simulink library "icc_lib_avg_path1_n1"  (R2018b)
settings: Solver=VariableStepAuto  StartTime=0.0  StopTime=10.0  RelTol=1e-3
undefined symbols (not defined in the file or in its folder): icc_lib_avg_path, path1
libraries: simulink x34, simulink_extras x8, $bdroot x2
(part 1 of 4)
settings Model: Creator=lwan353  LastModifiedBy=lwan353
settings SFSimCC: SimUseLocalCustomCode=off
settings RTWCC: RTWUseLocalCustomCode=off

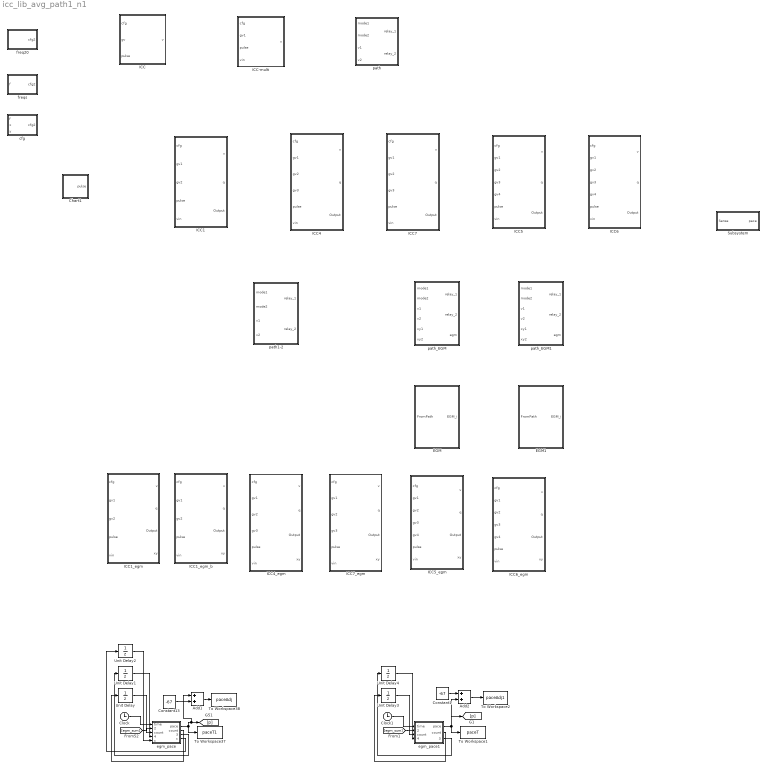
== system icc_lib_avg_path1_n1 ==
  Add1 : Sum
  Add2 : Sum
  Chart1 : Stateflow chart  TreatAsAtomicUnit=on
  Clock : Clock
  Clock1 : Clock
  Constant1 : Constant  Value=-67
  Constant13 : Constant  Value=-67
  EGM : Subsystem
  EGM1 : Subsystem
  "ICC " : Subsystem
  ICC-multi : Subsystem
  ICC1 : Subsystem
  ICC1_egm : Subsystem
  ICC1_egm_b : Subsystem
  ICC4 : Subsystem
  ICC4_egm : Subsystem
  ICC5 : Subsystem
  ICC5_egm : Subsystem
  ICC6 : Subsystem
  ICC6_egm : Subsystem
  ICC7 : Subsystem
  ICC7_egm : Subsystem
  Subsystem : Subsystem
  To Workspace1 : ToWorkspace  VariableName=paceT  SaveFormat=Timeseries  SampleTime=-1
  To Workspace2 : ToWorkspace  VariableName=paceAdj1  SaveFormat=Timeseries  SampleTime=-1
  To Workspace37 : ToWorkspace  VariableName=paceT1  SaveFormat=Timeseries  SampleTime=-1
  To Workspace38 : ToWorkspace  VariableName=paceAdj  SaveFormat=Timeseries  SampleTime=-1
  Unit Delay{,1..4} (5 alike) : UnitDelay  SampleTime=-1
  cfg : MATLAB Function  TreatAsAtomicUnit=on
  egm_pace : MATLAB Function  TreatAsAtomicUnit=on
  egm_pace1 : MATLAB Function  TreatAsAtomicUnit=on
  freq20 : MATLAB Function  TreatAsAtomicUnit=on
  freqs : MATLAB Function  TreatAsAtomicUnit=on
  path : Subsystem
  path1-2 : Subsystem  AncestorBlock=icc_lib_avg_path/path1
  path_EGM : Subsystem
  path_EGM1 : Subsystem
  wires:
  Unit Delay/1 -> egm_pace/3("count ")
  Clock/1 -> egm_pace/1(time)
  [egm_sum] -> egm_pace/2(egm_sum)
  egm_pace/2(count) -> Unit Delay/1
  egm_pace/1(pace) -> Add1/1, [p], To Workspace37/1
  Unit Delay2/1 -> egm_pace/5("c ")
  egm_pace/3(basetime) -> Unit Delay1/1
  Constant13/1 -> Add1/2
  Unit Delay1/1 -> egm_pace/4("basetime ")
  Add1/1 -> To Workspace38/1
  egm_pace/4(c) -> Unit Delay2/1
  Unit Delay3/1 -> egm_pace1/3("count ")
  Clock1/1 -> egm_pace1/1(time)
  [egm_sum] -> egm_pace1/2(egm_sum)
  egm_pace1/2(count) -> Unit Delay3/1
  egm_pace1/1(pace) -> [p], To Workspace1/1, Add2/2
  egm_pace1/3(basetime) -> Unit Delay4/1
  Constant1/1 -> Add2/1
  Unit Delay4/1 -> egm_pace1/4("basetime ")
  Add2/1 -> To Workspace2/1

== system icc_lib_avg_path1_n1/EGM ==
  FromPath : Inport
  Constant : Constant  Value=18
  Constant1 : Constant  Value=10
  Constant2 : Constant  Value=10
  Demux4 : Demux  Outputs=6
  Path2 : Stateflow chart  TreatAsAtomicUnit=on
  sum : Sum
  EGM_i : Outport
  wires:
  [yj] -> Path2/4(yj)
  [xj] -> Path2/3(xj)
  Constant1/1 -> Path2/5(cvi)
  [ti] -> Path2/7(t1)
  [tj] -> Path2/8(t2)
  Demux4/5 -> [xj]
  Demux4/4 -> [yi]
  FromPath/1 -> Demux4/1
  [xi] -> Path2/1(xi)
  Demux4/3 -> [xi]
  Path2/2(egm_j) -> sum/2
  sum/1 -> EGM_i/1
  Path2/1(egm_i) -> sum/1
  Constant/1 -> Path2/9(C)
  [yi] -> Path2/2(yi)
  Demux4/6 -> [yj]
  Constant2/1 -> Path2/6(cvj)
  Demux4/2 -> [tj]
  Demux4/1 -> [ti]

== system icc_lib_avg_path1_n1/EGM1 ==
  FromPath : Inport
  Constant : Constant  Value=18
  Constant1 : Constant  Value=6
  Constant2 : Constant  Value=6
  Demux4 : Demux  Outputs=6
  Path2 : Stateflow chart  TreatAsAtomicUnit=on
  sum : Sum
  EGM_i : Outport
  wires:
  [yj] -> Path2/4(yj)
  [xj] -> Path2/3(xj)
  Constant1/1 -> Path2/5(cvi)
  [ti] -> Path2/7(t1)
  [tj] -> Path2/8(t2)
  Demux4/5 -> [xj]
  Demux4/4 -> [yi]
  FromPath/1 -> Demux4/1
  [xi] -> Path2/1(xi)
  Demux4/3 -> [xi]
  Path2/2(egm_j) -> sum/2
  sum/1 -> EGM_i/1
  Path2/1(egm_i) -> sum/1
  Constant/1 -> Path2/9(C)
  [yi] -> Path2/2(yi)
  Demux4/6 -> [yj]
  Constant2/1 -> Path2/6(cvj)
  Demux4/2 -> [tj]
  Demux4/1 -> [ti]

== system icc_lib_avg_path1_n1/ICC  ==
  "cfg " : Inport
  gv : Inport  Port=2
  pulse : Inport  Port=3
  Add : Sum
  Chart : Stateflow chart  TreatAsAtomicUnit=on
  Chart1 : Stateflow chart  TreatAsAtomicUnit=on
  Constant : Constant  Value=0
  Demux : Demux  Outputs=8
  MATLAB Function : MATLAB Function  TreatAsAtomicUnit=on
  "MATLAB Function-freq=22 " : MATLAB Function  TreatAsAtomicUnit=on
  MATLAB Function-freq=24 : MATLAB Function  TreatAsAtomicUnit=on
  "MATLAB Function-freq=26 " : MATLAB Function  TreatAsAtomicUnit=on
  "MATLAB Function-freq=26-o " : MATLAB Function  TreatAsAtomicUnit=on
  "MATLAB Function1-freq=20 " : MATLAB Function  TreatAsAtomicUnit=on
  ODE : Subsystem
  v : Outport
  wires:
  [d3] -> ODE/6(d3)
  Demux/6 -> [Vm]
  Demux/1 -> [d0]
  Demux/4 -> [d3]
  Chart/2(vreset) -> ODE/2(vreset)
  Chart/1(q) -> ODE/1(q)
  [d0] -> ODE/3(d0)
  Demux/7 -> [VR]
  Chart/3(d2) -> ODE/5(d2)
  [VT] -> Chart/4(VT)
  ODE/1(vt_0) -> Chart/1(v), v/1
  Demux/3 -> [d2i]
  [VR] -> Chart/6(VR)
  [VF] -> Chart/7(VF)
  [d2i] -> Chart/8(d2i)
  Demux/2 -> [d1]
  Add/1 -> Chart/2(gv)
  Demux/5 -> [VT]
  "cfg "/1 -> Demux/1
  Chart/4(reset) -> ODE/7(reset)
  [Vm] -> Chart/5(Vm)
  [d1] -> ODE/4(d1)
  Demux/8 -> [VF]
  pulse/1 -> Add/1
  gv/1 -> Add/2

== system icc_lib_avg_path1_n1/ICC-multi ==
  "cfg " : Inport
  gv1 : Inport  Port=2
  pulse : Inport  Port=3
  vin : Inport  Port=4
  Add : Sum  Inputs=+-
  Add1 : Sum
  Chart : Stateflow chart  TreatAsAtomicUnit=on
  Constant1 : Constant  Value=0.2
  Constant2 : Constant  Value=1.25
  Demux : Demux  Outputs=8
  Divide1 : Product  CollapseMode=Specified dimension  CollapseDim=2  SaturateOnIntegerOverflow=on  RndMeth=Zero
  Divide2 : Product  CollapseMode=Specified dimension  CollapseDim=2  SaturateOnIntegerOverflow=on  RndMeth=Zero
  MATLAB Function : MATLAB Function  TreatAsAtomicUnit=on
  "MATLAB Function-freq=22 " : MATLAB Function  TreatAsAtomicUnit=on
  MATLAB Function-freq=24 : MATLAB Function  TreatAsAtomicUnit=on
  "MATLAB Function-freq=26 " : MATLAB Function  TreatAsAtomicUnit=on
  "MATLAB Function-freq=26-o " : MATLAB Function  TreatAsAtomicUnit=on
  "MATLAB Function1-freq=20 " : MATLAB Function  TreatAsAtomicUnit=on
  ODE : Subsystem
  v : Outport
  wires:
  Demux/6 -> [Vm]
  Demux/1 -> [d0]
  Demux/4 -> [d3]
  Demux/7 -> [VR]
  Demux/3 -> [d2i]
  Demux/2 -> [d1]
  Demux/5 -> [VT]
  "cfg "/1 -> Demux/1
  Demux/8 -> [VF]
  Divide2/1 -> Add/2
  [d3] -> ODE/6(d3)
  Add/1 -> Divide1/1
  ODE/1(vt_0) -> v/1, Chart/1(v)
  [VT] -> Chart/4(VT)
  Chart/3(d2) -> ODE/5(d2)
  [d0] -> ODE/3(d0)
  [d2i] -> Chart/8(d2i)
  pulse/1 -> Add1/1
  Chart/2(vreset) -> ODE/2(vreset)
  [VR] -> Chart/6(VR)
  Chart/1(q) -> ODE/1(q)
  [VF] -> Chart/7(VF)
  Constant2/1 -> Divide1/2
  Constant1/1 -> Divide2/2
  Chart/4(reset) -> ODE/7(reset)
  vin/1 -> Divide2/1
  Add1/1 -> Chart/2(gv)
  Divide1/1 -> Add1/2
  gv1/1 -> Add/1
  [Vm] -> Chart/5(Vm)
  [d1] -> ODE/4(d1)

== system icc_lib_avg_path1_n1/ICC1 ==
  "cfg " : Inport
  gv1 : Inport  Port=2
  gv2 : Inport  Port=3
  pulse : Inport  Port=4
  vin : Inport  Port=5
  Add : Sum  Inputs=+-
  Add1 : Sum
  Add2 : Sum  Inputs=+-
  Chart : Stateflow chart  TreatAsAtomicUnit=on
  Constant1 : Constant  Value=0.5
  Constant2 : Constant
  Constant3 : Constant  Value=-67
  Constant4 : Constant
  Constant5 : Constant  Value=-67
  Constant6 : Constant  Value=0
  Demux : Demux  Outputs=8
  Divide1 : Product  CollapseMode=Specified dimension  CollapseDim=2  SaturateOnIntegerOverflow=on  RndMeth=Zero
  Divide2 : Product  CollapseMode=Specified dimension  CollapseDim=2  SaturateOnIntegerOverflow=on  RndMeth=Zero
  Divide3 : Product  CollapseMode=Specified dimension  CollapseDim=2  SaturateOnIntegerOverflow=on  RndMeth=Zero
  MATLAB Function : MATLAB Function  TreatAsAtomicUnit=on
  "MATLAB Function-freq=22 " : MATLAB Function  TreatAsAtomicUnit=on
  MATLAB Function-freq=24 : MATLAB Function  TreatAsAtomicUnit=on
  "MATLAB Function-freq=26 " : MATLAB Function  TreatAsAtomicUnit=on
  "MATLAB Function-freq=26-o " : MATLAB Function  TreatAsAtomicUnit=on
  "MATLAB Function1-freq=20 " : MATLAB Function  TreatAsAtomicUnit=on
  Memory : Memory  InheritSampleTime=on
  Memory1 : Memory  InheritSampleTime=on
  ODE : Subsystem
  Sum : Sum  Inputs=|++
  v : Outport
  q : Outport  Port=2
  Output : Outport  Port=3
  wires:
  gv1/1 -> Add/1
  Divide1/1 -> Sum/1
  vin/1 -> Divide2/1
  Constant2/1 -> Divide1/2
  pulse/1 -> Add1/1
  Demux/8 -> [VF]
  [d1] -> ODE/4(d1)
  [Vm] -> Chart/4(Vm)
  Chart/5(reset) -> ODE/7(reset)
  "cfg "/1 -> Demux/1
  Demux/5 -> [VT]
  Add1/1 -> Chart/2(gv)
  Demux/2 -> [d1]
  [d2i] -> Chart/7(d2i)
  [VF] -> Chart/6(VF)
  [VR] -> Chart/5(VR)
  Demux/3 -> [d2i]
  ODE/1(vt_0) -> v/1, Chart/1(v)
  [VT] -> Chart/3(VT)
  Chart/3(d2) -> ODE/5(d2)
  Demux/7 -> [VR]
  [d0] -> ODE/3(d0)
  Chart/2(vreset) -> ODE/2(vreset)
  Demux/4 -> [d3]
  Demux/1 -> [d0]
  Demux/6 -> [Vm]
  [d3] -> ODE/6(d3)
  Constant1/1 -> Divide2/2
  Divide2/1 -> Add2/2, Add/2
  Add/1 -> Divide1/1
  Constant3/1 -> ?
  Chart/1(q) -> Memory/1
  Memory/1 -> ODE/1(q), q/1
  gv2/1 -> Add2/1
  Constant4/1 -> Divide3/2
  Divide3/1 -> Sum/2
  Add2/1 -> Divide3/1
  Sum/1 -> Add1/2
  Chart/4(Sense) -> Memory1/1
  Memory1/1 -> Output/1

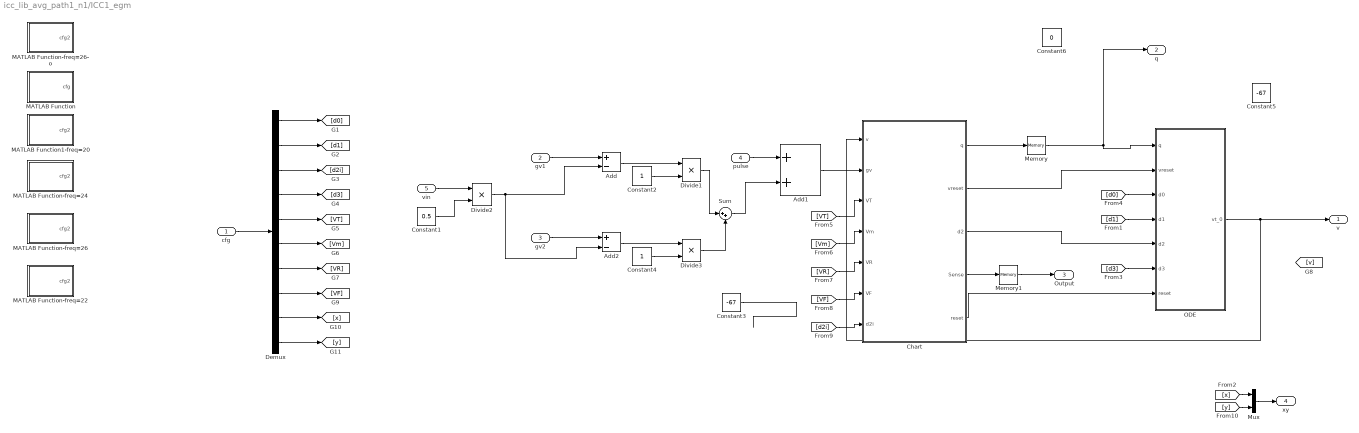
== system icc_lib_avg_path1_n1/ICC1_egm ==
  "cfg " : Inport
  gv1 : Inport  Port=2
  gv2 : Inport  Port=3
  pulse : Inport  Port=4
  vin : Inport  Port=5
  Add : Sum  Inputs=+-
  Add1 : Sum
  Add2 : Sum  Inputs=+-
  Chart : Stateflow chart  TreatAsAtomicUnit=on
  Constant1 : Constant  Value=0.5
  Constant2 : Constant
  Constant3 : Constant  Value=-67
  Constant4 : Constant
  Constant5 : Constant  Value=-67
  Constant6 : Constant  Value=0
  Demux : Demux  Outputs=10
  Divide1 : Product  CollapseMode=Specified dimension  CollapseDim=2  SaturateOnIntegerOverflow=on  RndMeth=Zero
  Divide2 : Product  CollapseMode=Specified dimension  CollapseDim=2  SaturateOnIntegerOverflow=on  RndMeth=Zero
  Divide3 : Product  CollapseMode=Specified dimension  CollapseDim=2  SaturateOnIntegerOverflow=on  RndMeth=Zero
  MATLAB Function : MATLAB Function  TreatAsAtomicUnit=on
  "MATLAB Function-freq=22 " : MATLAB Function  TreatAsAtomicUnit=on
  MATLAB Function-freq=24 : MATLAB Function  TreatAsAtomicUnit=on
  "MATLAB Function-freq=26 " : MATLAB Function  TreatAsAtomicUnit=on
  "MATLAB Function-freq=26-o " : MATLAB Function  TreatAsAtomicUnit=on
  "MATLAB Function1-freq=20 " : MATLAB Function  TreatAsAtomicUnit=on
  Memory : Memory  InheritSampleTime=on
  Memory1 : Memory  InheritSampleTime=on
  Mux : Mux  Inputs=2
  ODE : Subsystem
  Sum : Sum  Inputs=|++
  v : Outport
  q : Outport  Port=2
  Output : Outport  Port=3
  xy : Outport  Port=4
  wires:
  gv1/1 -> Add/1
  Divide1/1 -> Sum/1
  vin/1 -> Divide2/1
  Constant2/1 -> Divide1/2
  pulse/1 -> Add1/1
  Demux/8 -> [VF]
  [d1] -> ODE/4(d1)
  [Vm] -> Chart/4(Vm)
  Chart/5(reset) -> ODE/7(reset)
  "cfg "/1 -> Demux/1
  Demux/5 -> [VT]
  Add1/1 -> Chart/2(gv)
  Demux/2 -> [d1]
  [d2i] -> Chart/7(d2i)
  [VF] -> Chart/6(VF)
  [VR] -> Chart/5(VR)
  Demux/3 -> [d2i]
  ODE/1(vt_0) -> v/1, Chart/1(v)
  [VT] -> Chart/3(VT)
  Chart/3(d2) -> ODE/5(d2)
  Demux/7 -> [VR]
  [d0] -> ODE/3(d0)
  Chart/2(vreset) -> ODE/2(vreset)
  Demux/4 -> [d3]
  Demux/1 -> [d0]
  Demux/6 -> [Vm]
  [d3] -> ODE/6(d3)
  Constant1/1 -> Divide2/2
  Divide2/1 -> Add2/2, Add/2
  Add/1 -> Divide1/1
  Constant3/1 -> ?
  Chart/1(q) -> Memory/1
  Memory/1 -> ODE/1(q), q/1
  gv2/1 -> Add2/1
  Constant4/1 -> Divide3/2
  Divide3/1 -> Sum/2
  Add2/1 -> Divide3/1
  Sum/1 -> Add1/2
  Chart/4(Sense) -> Memory1/1
  Memory1/1 -> Output/1
  Demux/9 -> [x]
  Demux/10 -> [y]
  Mux/1 -> xy/1
  [x] -> Mux/1
  [y] -> Mux/2

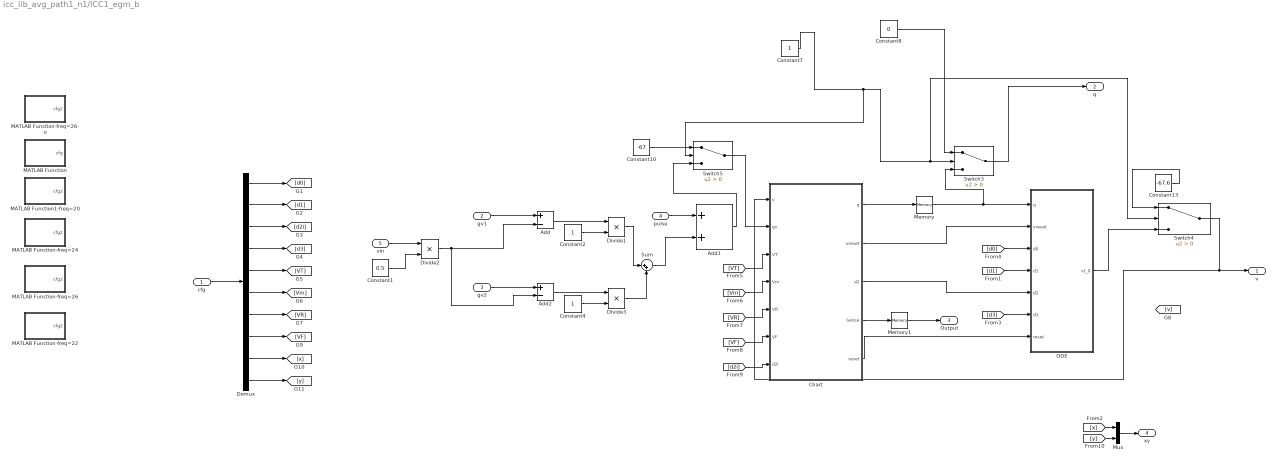
== system icc_lib_avg_path1_n1/ICC1_egm_b ==
  "cfg " : Inport
  gv1 : Inport  Port=2
  gv2 : Inport  Port=3
  pulse : Inport  Port=4
  vin : Inport  Port=5
  Add : Sum  Inputs=+-
  Add1 : Sum
  Add2 : Sum  Inputs=+-
  Chart : Stateflow chart  TreatAsAtomicUnit=on
  Constant1 : Constant  Value=0.5
  Constant10 : Constant  Value=-67
  Constant13 : Constant  Value=-67.6
  Constant2 : Constant
  Constant4 : Constant
  Constant7 : Constant
  Constant8 : Constant  Value=0
  Demux : Demux  Outputs=10
  Divide1 : Product  CollapseMode=Specified dimension  CollapseDim=2  SaturateOnIntegerOverflow=on  RndMeth=Zero
  Divide2 : Product  CollapseMode=Specified dimension  CollapseDim=2  SaturateOnIntegerOverflow=on  RndMeth=Zero
  Divide3 : Product  CollapseMode=Specified dimension  CollapseDim=2  SaturateOnIntegerOverflow=on  RndMeth=Zero
  MATLAB Function : MATLAB Function  TreatAsAtomicUnit=on
  "MATLAB Function-freq=22 " : MATLAB Function  TreatAsAtomicUnit=on
  MATLAB Function-freq=24 : MATLAB Function  TreatAsAtomicUnit=on
  "MATLAB Function-freq=26 " : MATLAB Function  TreatAsAtomicUnit=on
  "MATLAB Function-freq=26-o " : MATLAB Function  TreatAsAtomicUnit=on
  "MATLAB Function1-freq=20 " : MATLAB Function  TreatAsAtomicUnit=on
  Memory : Memory  InheritSampleTime=on
  Memory1 : Memory  InheritSampleTime=on
  Mux : Mux  Inputs=2
  ODE : Subsystem
  Sum : Sum  Inputs=|++
  Switch3 : Switch  Criteria=u2 > Threshold
  Switch4 : Switch  Criteria=u2 > Threshold
  Switch5 : Switch  Criteria=u2 > Threshold
  v : Outport
  q : Outport  Port=2
  Output : Outport  Port=3
  xy : Outport  Port=4
  wires:
  gv1/1 -> Add/1
  Divide1/1 -> Sum/1
  vin/1 -> Divide2/1
  Constant2/1 -> Divide1/2
  pulse/1 -> Add1/1
  Demux/8 -> [VF]
  [d1] -> ODE/4(d1)
  [Vm] -> Chart/4(Vm)
  Chart/5(reset) -> ODE/7(reset)
  "cfg "/1 -> Demux/1
  Demux/5 -> [VT]
  Demux/2 -> [d1]
  [d2i] -> Chart/7(d2i)
  [VF] -> Chart/6(VF)
  [VR] -> Chart/5(VR)
  Demux/3 -> [d2i]
  Switch4/1 -> Chart/1(v), v/1
  [VT] -> Chart/3(VT)
  Chart/3(d2) -> ODE/5(d2)
  Demux/7 -> [VR]
  [d0] -> ODE/3(d0)
  Chart/2(vreset) -> ODE/2(vreset)
  Demux/4 -> [d3]
  Demux/1 -> [d0]
  Demux/6 -> [Vm]
  [d3] -> ODE/6(d3)
  Constant1/1 -> Divide2/2
  Divide2/1 -> Add2/2, Add/2
  Add/1 -> Divide1/1
  Chart/1(q) -> Memory/1
  gv2/1 -> Add2/1
  Constant4/1 -> Divide3/2
  Divide3/1 -> Sum/2
  Add2/1 -> Divide3/1
  Sum/1 -> Add1/2
  Chart/4(Sense) -> Memory1/1
  Memory1/1 -> Output/1
  Demux/9 -> [x]
  Demux/10 -> [y]
  Mux/1 -> xy/1
  [x] -> Mux/1
  [y] -> Mux/2
  Switch5/1 -> Chart/2(gv)
  Constant8/1 -> Switch3/1
  Constant10/1 -> Switch5/1
  Add1/1 -> Switch5/3
  Constant7/1 -> Switch4/2, Switch3/2, Switch5/2
  Constant13/1 -> Switch4/1
  Memory/1 -> Switch3/3, ODE/1(q)
  Switch3/1 -> q/1
  ODE/1(vt_0) -> Switch4/3

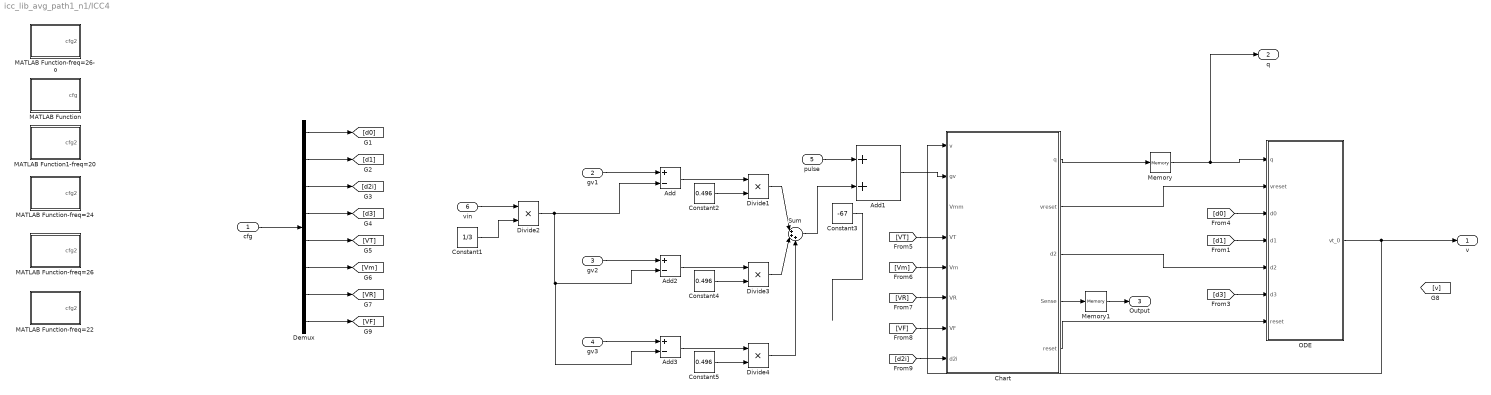
== system icc_lib_avg_path1_n1/ICC4 ==
  "cfg " : Inport
  gv1 : Inport  Port=2
  gv2 : Inport  Port=3
  gv3 : Inport  Port=4
  pulse : Inport  Port=5
  vin : Inport  Port=6
  Add : Sum  Inputs=+-
  Add1 : Sum
  Add2 : Sum  Inputs=+-
  Add3 : Sum  Inputs=+-
  Chart : Stateflow chart  TreatAsAtomicUnit=on
  Constant1 : Constant  Value=1/3
  Constant2 : Constant  Value=0.496
  Constant3 : Constant  Value=-67
  Constant4 : Constant  Value=0.496
  Constant5 : Constant  Value=0.496
  Demux : Demux  Outputs=8
  Divide{1..4} (4 alike) : Product  CollapseMode=Specified dimension  CollapseDim=2  SaturateOnIntegerOverflow=on  RndMeth=Zero
  MATLAB Function : MATLAB Function  TreatAsAtomicUnit=on
  "MATLAB Function-freq=22 " : MATLAB Function  TreatAsAtomicUnit=on
  MATLAB Function-freq=24 : MATLAB Function  TreatAsAtomicUnit=on
  "MATLAB Function-freq=26 " : MATLAB Function  TreatAsAtomicUnit=on
  "MATLAB Function-freq=26-o " : MATLAB Function  TreatAsAtomicUnit=on
  "MATLAB Function1-freq=20 " : MATLAB Function  TreatAsAtomicUnit=on
  Memory : Memory  InheritSampleTime=on
  Memory1 : Memory  InheritSampleTime=on
  ODE : Subsystem
  Sum : Sum  Inputs=|+++
  v : Outport
  q : Outport  Port=2
  Output : Outport  Port=3
  wires:
  Chart/4(Sense) -> Memory1/1
  Constant5/1 -> Divide4/2
  [d2i] -> Chart/8(d2i)
  Constant4/1 -> Divide3/2
  Divide4/1 -> Sum/3
  Add2/1 -> Divide3/1
  [VT] -> Chart/4(VT)
  Demux/3 -> [d2i]
  [VR] -> Chart/6(VR)
  gv2/1 -> Add2/1
  Memory/1 -> q/1, ODE/1(q)
  Demux/4 -> [d3]
  Demux/1 -> [d0]
  Add/1 -> Divide1/1
  Constant2/1 -> Divide1/2
  Chart/3(d2) -> ODE/5(d2)
  Chart/2(vreset) -> ODE/2(vreset)
  vin/1 -> Divide2/1
  [d3] -> ODE/6(d3)
  pulse/1 -> Add1/1
  Add3/1 -> Divide4/1
  Chart/5(reset) -> ODE/7(reset)
  ODE/1(vt_0) -> v/1, Chart/1(v)
  Constant1/1 -> Divide2/2
  gv3/1 -> Add3/1
  Divide1/1 -> Sum/1
  Divide3/1 -> Sum/2
  [Vm] -> Chart/5(Vm)
  [d0] -> ODE/3(d0)
  [VF] -> Chart/7(VF)
  Sum/1 -> Add1/2
  Add1/1 -> Chart/2(gv)
  Memory1/1 -> Output/1
  Divide2/1 -> Add2/2, Add3/2, Add/2
  gv1/1 -> Add/1
  Demux/5 -> [VT]
  Demux/8 -> [VF]
  "cfg "/1 -> Demux/1
  Demux/7 -> [VR]
  Demux/2 -> [d1]
  Demux/6 -> [Vm]
  Constant3/1 -> ?
  [d1] -> ODE/4(d1)
  Chart/1(q) -> Memory/1

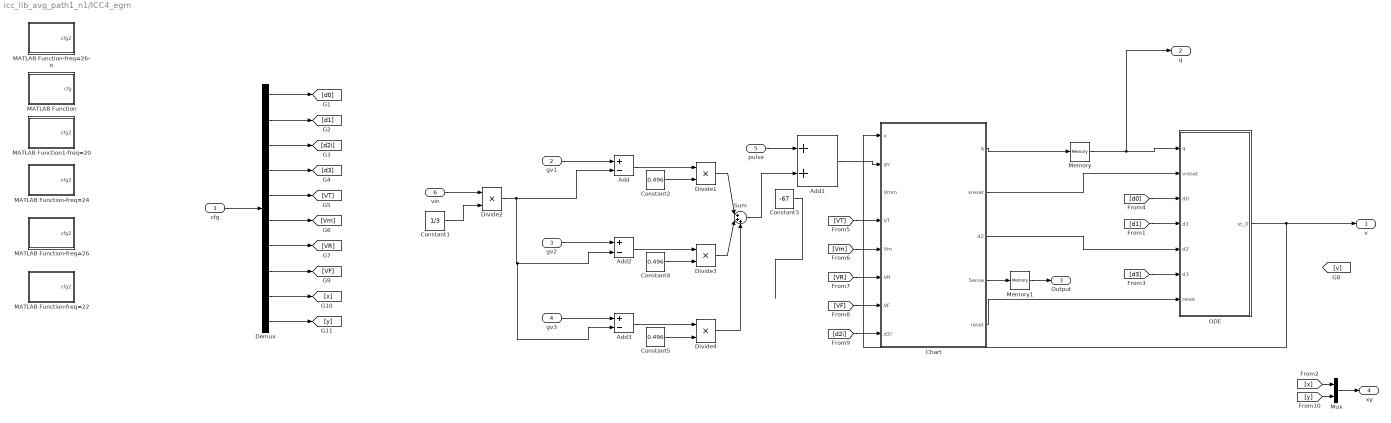
== system icc_lib_avg_path1_n1/ICC4_egm ==
  "cfg " : Inport
  gv1 : Inport  Port=2
  gv2 : Inport  Port=3
  gv3 : Inport  Port=4
  pulse : Inport  Port=5
  vin : Inport  Port=6
  Add : Sum  Inputs=+-
  Add1 : Sum
  Add2 : Sum  Inputs=+-
  Add3 : Sum  Inputs=+-
  Chart : Stateflow chart  TreatAsAtomicUnit=on
  Constant1 : Constant  Value=1/3
  Constant2 : Constant  Value=0.496
  Constant3 : Constant  Value=-67
  Constant4 : Constant  Value=0.496
  Constant5 : Constant  Value=0.496
  Demux : Demux  Outputs=10
  Divide{1..4} (4 alike) : Product  CollapseMode=Specified dimension  CollapseDim=2  SaturateOnIntegerOverflow=on  RndMeth=Zero
  MATLAB Function : MATLAB Function  TreatAsAtomicUnit=on
  "MATLAB Function-freq=22 " : MATLAB Function  TreatAsAtomicUnit=on
  MATLAB Function-freq=24 : MATLAB Function  TreatAsAtomicUnit=on
  "MATLAB Function-freq=26 " : MATLAB Function  TreatAsAtomicUnit=on
  "MATLAB Function-freq=26-o " : MATLAB Function  TreatAsAtomicUnit=on
  "MATLAB Function1-freq=20 " : MATLAB Function  TreatAsAtomicUnit=on
  Memory : Memory  InheritSampleTime=on
  Memory1 : Memory  InheritSampleTime=on
  Mux : Mux  Inputs=2
  ODE : Subsystem
  Sum : Sum  Inputs=|+++
  v : Outport
  q : Outport  Port=2
  Output : Outport  Port=3
  xy : Outport  Port=4
  wires:
  Chart/4(Sense) -> Memory1/1
  Constant5/1 -> Divide4/2
  [d2i] -> Chart/8(d2i)
  Constant4/1 -> Divide3/2
  Divide4/1 -> Sum/3
  Add2/1 -> Divide3/1
  [VT] -> Chart/4(VT)
  [VR] -> Chart/6(VR)
  gv2/1 -> Add2/1
  Memory/1 -> q/1, ODE/1(q)
  Add/1 -> Divide1/1
  Constant2/1 -> Divide1/2
  Chart/3(d2) -> ODE/5(d2)
  Chart/2(vreset) -> ODE/2(vreset)
  vin/1 -> Divide2/1
  [d3] -> ODE/6(d3)
  pulse/1 -> Add1/1
  Add3/1 -> Divide4/1
  Chart/5(reset) -> ODE/7(reset)
  ODE/1(vt_0) -> v/1, Chart/1(v)
  Constant1/1 -> Divide2/2
  gv3/1 -> Add3/1
  Divide1/1 -> Sum/1
  Divide3/1 -> Sum/2
  [Vm] -> Chart/5(Vm)
  [d0] -> ODE/3(d0)
  [VF] -> Chart/7(VF)
  Sum/1 -> Add1/2
  Add1/1 -> Chart/2(gv)
  Memory1/1 -> Output/1
  Divide2/1 -> Add2/2, Add3/2, Add/2
  gv1/1 -> Add/1
  Constant3/1 -> ?
  [d1] -> ODE/4(d1)
  Chart/1(q) -> Memory/1
  "cfg "/1 -> Demux/1
  Demux/8 -> [VF]
  Demux/4 -> [d3]
  Demux/2 -> [d1]
  Demux/3 -> [d2i]
  Demux/5 -> [VT]
  Demux/9 -> [x]
  Demux/1 -> [d0]
  Demux/7 -> [VR]
  Demux/10 -> [y]
  Demux/6 -> [Vm]
  [x] -> Mux/1
  [y] -> Mux/2
  Mux/1 -> xy/1

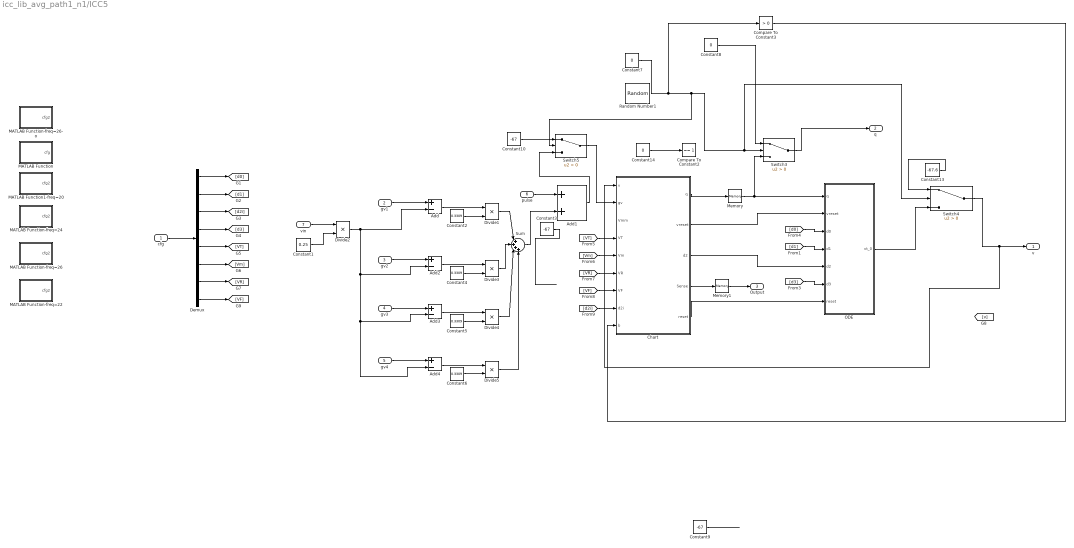
== system icc_lib_avg_path1_n1/ICC5 ==
  "cfg " : Inport
  gv1 : Inport  Port=2
  gv2 : Inport  Port=3
  gv3 : Inport  Port=4
  gv4 : Inport  Port=5
  pulse : Inport  Port=6
  vin : Inport  Port=7
  Add{,2..4} (4 alike) : Sum  Inputs=+-
  Add1 : Sum
  Chart : Stateflow chart  TreatAsAtomicUnit=on
  Compare To Constant2 : simulink/Logic and Bit Operations/Compare To Constant  relop===  const=1  OutDataTypeStr=boolean
  Compare To Constant3 : simulink/Logic and Bit Operations/Compare To Constant  relop=>  const=0  OutDataTypeStr=boolean
  Constant1 : Constant  Value=0.25
  Constant10 : Constant  Value=-67
  Constant13 : Constant  Value=-67.6
  Constant14 : Constant  Value=0
  Constant{2,4..6} (4 alike) : Constant  Value=0.3309
  Constant3 : Constant  Value=-67
  Constant7 : Constant  Value=0
  Constant8 : Constant  Value=0
  Constant9 : Constant  Value=-67
  Demux : Demux  Outputs=8
  Divide{1..5} (5 alike) : Product  CollapseMode=Specified dimension  CollapseDim=2  SaturateOnIntegerOverflow=on  RndMeth=Zero
  MATLAB Function : MATLAB Function  TreatAsAtomicUnit=on
  "MATLAB Function-freq=22 " : MATLAB Function  TreatAsAtomicUnit=on
  MATLAB Function-freq=24 : MATLAB Function  TreatAsAtomicUnit=on
  "MATLAB Function-freq=26 " : MATLAB Function  TreatAsAtomicUnit=on
  "MATLAB Function-freq=26-o " : MATLAB Function  TreatAsAtomicUnit=on
  "MATLAB Function1-freq=20 " : MATLAB Function  TreatAsAtomicUnit=on
  Memory : Memory  InheritSampleTime=on
  Memory1 : Memory  InheritSampleTime=on
  ODE : Subsystem
  Random Number1 : RandomNumber  SampleTime=20.2
  Sum : Sum  Inputs=|++++
  Switch3 : Switch  Criteria=u2 > Threshold
  Switch4 : Switch  Criteria=u2 > Threshold
  Switch5 : Switch  Criteria=u2 > Threshold
  v : Outport
  q : Outport  Port=2
  Output : Outport  Port=3
  wires:
  gv1/1 -> Add/1
  Divide1/1 -> Sum/1
  vin/1 -> Divide2/1
  Constant2/1 -> Divide1/2
  pulse/1 -> Add1/1
  Demux/8 -> [VF]
  "cfg "/1 -> Demux/1
  Demux/5 -> [VT]
  Demux/2 -> [d1]
  Demux/3 -> [d2i]
  Demux/7 -> [VR]
  Demux/4 -> [d3]
  Demux/1 -> [d0]
  Demux/6 -> [Vm]
  Constant1/1 -> Divide2/2
  Add/1 -> Divide1/1
  Constant3/1 -> ?
  gv2/1 -> Add2/1
  Constant4/1 -> Divide3/2
  Divide3/1 -> Sum/2
  Add2/1 -> Divide3/1
  Sum/1 -> Add1/2
  Add3/1 -> Divide4/1
  Constant5/1 -> Divide4/2
  gv3/1 -> Add3/1
  Divide2/1 -> Add4/2, Add3/2, Add2/2, Add/2
  Add4/1 -> Divide5/1
  Constant6/1 -> Divide5/2
  Divide5/1 -> Sum/4
  gv4/1 -> Add4/1
  Divide4/1 -> Sum/3
  Constant7/1 -> Compare To Constant3/1, Switch5/2, Switch4/2, Switch3/2
  Switch4/1 -> Chart/1(v), v/1
  [d3] -> ODE/6(d3)
  [d1] -> ODE/4(d1)
  Chart/5(reset) -> ODE/7(reset)
  [VT] -> Chart/4(VT)
  [Vm] -> Chart/5(Vm)
  [VR] -> Chart/6(VR)
  Chart/3(d2) -> ODE/5(d2)
  Constant14/1 -> Compare To Constant2/1
  Add1/1 -> Switch5/3
  ODE/1(vt_0) -> Switch4/3
  [VF] -> Chart/7(VF)
  [d2i] -> Chart/8(d2i)
  Chart/1(q) -> Memory/1
  Switch5/1 -> Chart/2(gv)
  Constant13/1 -> Switch4/1
  Memory/1 -> ODE/1(q), Switch3/3
  Switch3/1 -> q/1
  Compare To Constant3/1 -> Chart/9(b)
  Constant8/1 -> Switch3/1
  Chart/2(vreset) -> ODE/2(vreset)
  [d0] -> ODE/3(d0)
  Constant9/1 -> ?
  Constant10/1 -> Switch5/1
  Chart/4(Sense) -> Memory1/1
  Memory1/1 -> Output/1

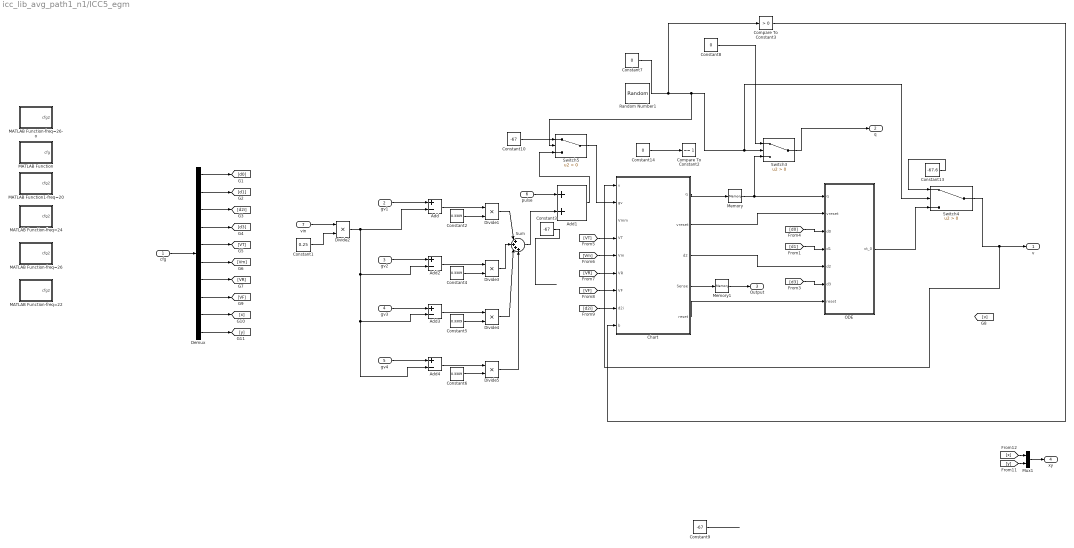
== system icc_lib_avg_path1_n1/ICC5_egm ==
  "cfg " : Inport
  gv1 : Inport  Port=2
  gv2 : Inport  Port=3
  gv3 : Inport  Port=4
  gv4 : Inport  Port=5
  pulse : Inport  Port=6
  vin : Inport  Port=7
  Add{,2..4} (4 alike) : Sum  Inputs=+-
  Add1 : Sum
  Chart : Stateflow chart  TreatAsAtomicUnit=on
  Compare To Constant2 : simulink/Logic and Bit Operations/Compare To Constant  relop===  const=1  OutDataTypeStr=boolean
  Compare To Constant3 : simulink/Logic and Bit Operations/Compare To Constant  relop=>  const=0  OutDataTypeStr=boolean
  Constant1 : Constant  Value=0.25
  Constant10 : Constant  Value=-67
  Constant13 : Constant  Value=-67.6
  Constant14 : Constant  Value=0
  Constant{2,4..6} (4 alike) : Constant  Value=0.3309
  Constant3 : Constant  Value=-67
  Constant7 : Constant  Value=0
  Constant8 : Constant  Value=0
  Constant9 : Constant  Value=-67
  Demux : Demux  Outputs=10
  Divide{1..5} (5 alike) : Product  CollapseMode=Specified dimension  CollapseDim=2  SaturateOnIntegerOverflow=on  RndMeth=Zero
  MATLAB Function : MATLAB Function  TreatAsAtomicUnit=on
  "MATLAB Function-freq=22 " : MATLAB Function  TreatAsAtomicUnit=on
  MATLAB Function-freq=24 : MATLAB Function  TreatAsAtomicUnit=on
  "MATLAB Function-freq=26 " : MATLAB Function  TreatAsAtomicUnit=on
  "MATLAB Function-freq=26-o " : MATLAB Function  TreatAsAtomicUnit=on
  "MATLAB Function1-freq=20 " : MATLAB Function  TreatAsAtomicUnit=on
  Memory : Memory  InheritSampleTime=on
  Memory1 : Memory  InheritSampleTime=on
  Mux1 : Mux  Inputs=2
  ODE : Subsystem
  Random Number1 : RandomNumber  SampleTime=20.2
  Sum : Sum  Inputs=|++++
  Switch3 : Switch  Criteria=u2 > Threshold
  Switch4 : Switch  Criteria=u2 > Threshold
  Switch5 : Switch  Criteria=u2 > Threshold
  v : Outport
  q : Outport  Port=2
  Output : Outport  Port=3
  xy : Outport  Port=4
  wires:
  gv1/1 -> Add/1
  Divide1/1 -> Sum/1
  vin/1 -> Divide2/1
  Constant2/1 -> Divide1/2
  pulse/1 -> Add1/1
  Constant1/1 -> Divide2/2
  Add/1 -> Divide1/1
  Constant3/1 -> ?
  gv2/1 -> Add2/1
  Constant4/1 -> Divide3/2
  Divide3/1 -> Sum/2
  Add2/1 -> Divide3/1
  Sum/1 -> Add1/2
  Add3/1 -> Divide4/1
  Constant5/1 -> Divide4/2
  gv3/1 -> Add3/1
  Divide2/1 -> Add4/2, Add3/2, Add2/2, Add/2
  Add4/1 -> Divide5/1
  Constant6/1 -> Divide5/2
  Divide5/1 -> Sum/4
  gv4/1 -> Add4/1
  Divide4/1 -> Sum/3
  Constant7/1 -> Compare To Constant3/1, Switch5/2, Switch4/2, Switch3/2
  Switch4/1 -> Chart/1(v), v/1
  [d3] -> ODE/6(d3)
  [d1] -> ODE/4(d1)
  Chart/5(reset) -> ODE/7(reset)
  [VT] -> Chart/4(VT)
  [Vm] -> Chart/5(Vm)
  [VR] -> Chart/6(VR)
  Chart/3(d2) -> ODE/5(d2)
  Constant14/1 -> Compare To Constant2/1
  Add1/1 -> Switch5/3
  ODE/1(vt_0) -> Switch4/3
  [VF] -> Chart/7(VF)
  [d2i] -> Chart/8(d2i)
  Chart/1(q) -> Memory/1
  Switch5/1 -> Chart/2(gv)
  Constant13/1 -> Switch4/1
  Memory/1 -> ODE/1(q), Switch3/3
  Switch3/1 -> q/1
  Compare To Constant3/1 -> Chart/9(b)
  Constant8/1 -> Switch3/1
  Chart/2(vreset) -> ODE/2(vreset)
  [d0] -> ODE/3(d0)
  Constant9/1 -> ?
  Constant10/1 -> Switch5/1
  Chart/4(Sense) -> Memory1/1
  Memory1/1 -> Output/1
  "cfg "/1 -> Demux/1
  Demux/8 -> [VF]
  Demux/4 -> [d3]
  Demux/2 -> [d1]
  Demux/3 -> [d2i]
  Demux/5 -> [VT]
  Demux/9 -> [x]
  Demux/1 -> [d0]
  Demux/7 -> [VR]
  Demux/10 -> [y]
  Demux/6 -> [Vm]
  [x] -> Mux1/1
  [y] -> Mux1/2
  Mux1/1 -> xy/1

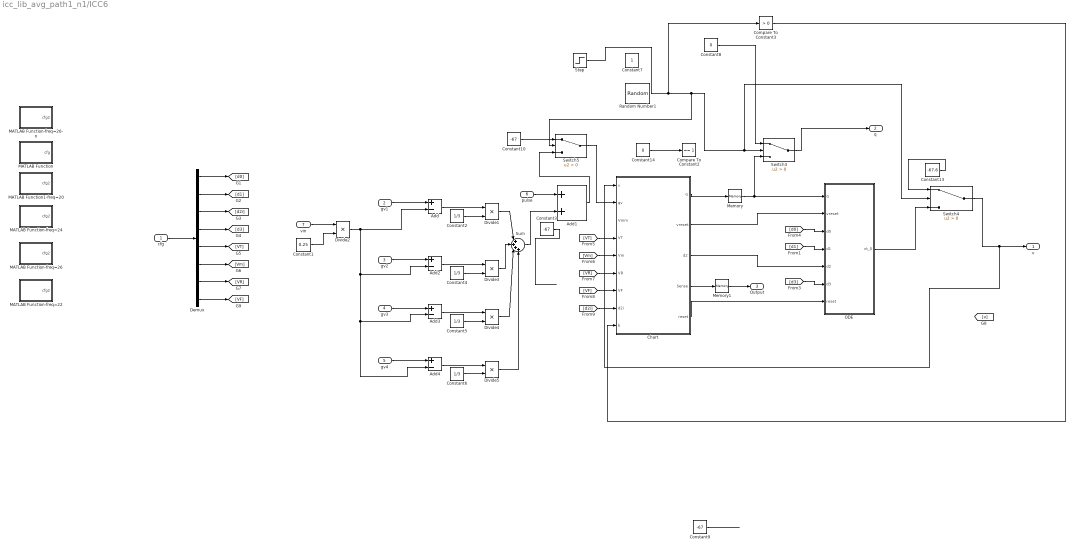
== system icc_lib_avg_path1_n1/ICC6 ==
  "cfg " : Inport
  gv1 : Inport  Port=2
  gv2 : Inport  Port=3
  gv3 : Inport  Port=4
  gv4 : Inport  Port=5
  pulse : Inport  Port=6
  vin : Inport  Port=7
  Add{,2..4} (4 alike) : Sum  Inputs=+-
  Add1 : Sum
  Chart : Stateflow chart  TreatAsAtomicUnit=on
  Compare To Constant2 : simulink/Logic and Bit Operations/Compare To Constant  relop===  const=1  OutDataTypeStr=boolean
  Compare To Constant3 : simulink/Logic and Bit Operations/Compare To Constant  relop=>  const=0  OutDataTypeStr=boolean
  Constant1 : Constant  Value=0.25
  Constant10 : Constant  Value=-67
  Constant13 : Constant  Value=-67.6
  Constant14 : Constant  Value=0
  Constant{2,4..6} (4 alike) : Constant  Value=1/3
  Constant3 : Constant  Value=-67
  Constant7 : Constant
  Constant8 : Constant  Value=0
  Constant9 : Constant  Value=-67
  Demux : Demux  Outputs=8
  Divide{1..5} (5 alike) : Product  CollapseMode=Specified dimension  CollapseDim=2  SaturateOnIntegerOverflow=on  RndMeth=Zero
  MATLAB Function : MATLAB Function  TreatAsAtomicUnit=on
  "MATLAB Function-freq=22 " : MATLAB Function  TreatAsAtomicUnit=on
  MATLAB Function-freq=24 : MATLAB Function  TreatAsAtomicUnit=on
  "MATLAB Function-freq=26 " : MATLAB Function  TreatAsAtomicUnit=on
  "MATLAB Function-freq=26-o " : MATLAB Function  TreatAsAtomicUnit=on
  "MATLAB Function1-freq=20 " : MATLAB Function  TreatAsAtomicUnit=on
  Memory : Memory  InheritSampleTime=on
  Memory1 : Memory  InheritSampleTime=on
  ODE : Subsystem
  Random Number1 : RandomNumber  SampleTime=20.2
  Step : Step  Time=52  Before=1  After=0  SampleTime=1
  Sum : Sum  Inputs=|++++
  Switch3 : Switch  Criteria=u2 > Threshold
  Switch4 : Switch  Criteria=u2 > Threshold
  Switch5 : Switch  Criteria=u2 > Threshold
  v : Outport
  q : Outport  Port=2
  Output : Outport  Port=3
  wires:
  gv1/1 -> Add/1
  Divide1/1 -> Sum/1
  vin/1 -> Divide2/1
  Constant2/1 -> Divide1/2
  pulse/1 -> Add1/1
  Demux/8 -> [VF]
  "cfg "/1 -> Demux/1
  Demux/5 -> [VT]
  Demux/2 -> [d1]
  Demux/3 -> [d2i]
  Demux/7 -> [VR]
  Demux/4 -> [d3]
  Demux/1 -> [d0]
  Demux/6 -> [Vm]
  Constant1/1 -> Divide2/2
  Add/1 -> Divide1/1
  Constant3/1 -> ?
  gv2/1 -> Add2/1
  Constant4/1 -> Divide3/2
  Divide3/1 -> Sum/2
  Add2/1 -> Divide3/1
  Sum/1 -> Add1/2
  Add3/1 -> Divide4/1
  Constant5/1 -> Divide4/2
  gv3/1 -> Add3/1
  Divide2/1 -> Add4/2, Add3/2, Add2/2, Add/2
  Add4/1 -> Divide5/1
  Constant6/1 -> Divide5/2
  Divide5/1 -> Sum/4
  gv4/1 -> Add4/1
  Divide4/1 -> Sum/3
  Step/1 -> Compare To Constant3/1, Switch5/2, Switch4/2, Switch3/2
  Switch4/1 -> Chart/1(v), v/1
  [d3] -> ODE/6(d3)
  [d1] -> ODE/4(d1)
  Chart/5(reset) -> ODE/7(reset)
  [VT] -> Chart/4(VT)
  [Vm] -> Chart/5(Vm)
  [VR] -> Chart/6(VR)
  Chart/3(d2) -> ODE/5(d2)
  Constant14/1 -> Compare To Constant2/1
  Add1/1 -> Switch5/3
  ODE/1(vt_0) -> Switch4/3
  [VF] -> Chart/7(VF)
  [d2i] -> Chart/8(d2i)
  Chart/1(q) -> Memory/1
  Switch5/1 -> Chart/2(gv)
  Constant13/1 -> Switch4/1
  Memory/1 -> ODE/1(q), Switch3/3
  Switch3/1 -> q/1
  Compare To Constant3/1 -> Chart/9(b)
  Constant8/1 -> Switch3/1
  Chart/2(vreset) -> ODE/2(vreset)
  [d0] -> ODE/3(d0)
  Constant9/1 -> ?
  Constant10/1 -> Switch5/1
  Chart/4(Sense) -> Memory1/1
  Memory1/1 -> Output/1

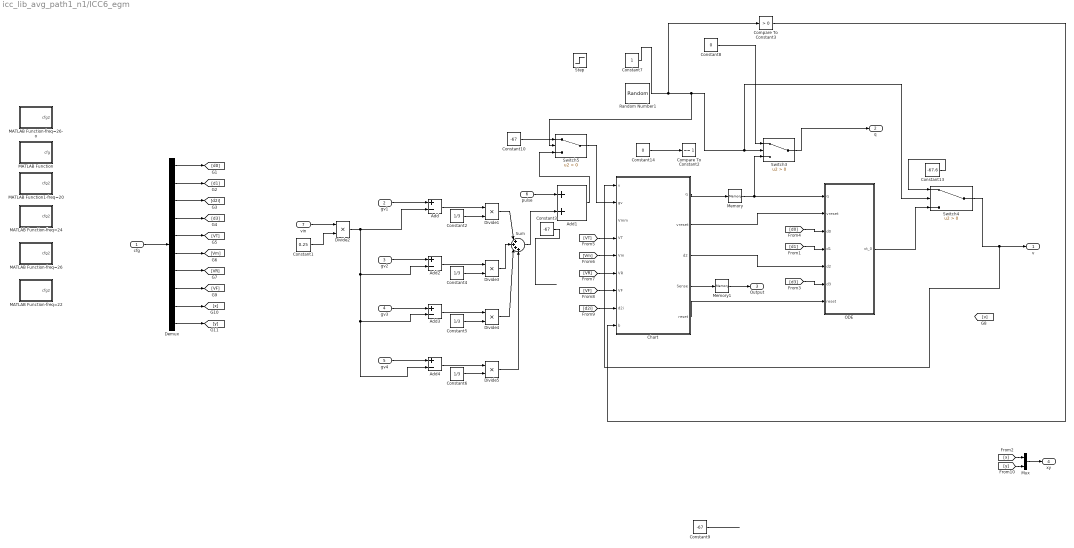
== system icc_lib_avg_path1_n1/ICC6_egm ==
  "cfg " : Inport
  gv1 : Inport  Port=2
  gv2 : Inport  Port=3
  gv3 : Inport  Port=4
  gv4 : Inport  Port=5
  pulse : Inport  Port=6
  vin : Inport  Port=7
  Add{,2..4} (4 alike) : Sum  Inputs=+-
  Add1 : Sum
  Chart : Stateflow chart  TreatAsAtomicUnit=on
  Compare To Constant2 : simulink/Logic and Bit Operations/Compare To Constant  relop===  const=1  OutDataTypeStr=boolean
  Compare To Constant3 : simulink/Logic and Bit Operations/Compare To Constant  relop=>  const=0  OutDataTypeStr=boolean
  Constant1 : Constant  Value=0.25
  Constant10 : Constant  Value=-67
  Constant13 : Constant  Value=-67.6
  Constant14 : Constant  Value=0
  Constant{2,4..6} (4 alike) : Constant  Value=1/3
  Constant3 : Constant  Value=-67
  Constant7 : Constant
  Constant8 : Constant  Value=0
  Constant9 : Constant  Value=-67
  Demux : Demux  Outputs=10
  Divide{1..5} (5 alike) : Product  CollapseMode=Specified dimension  CollapseDim=2  SaturateOnIntegerOverflow=on  RndMeth=Zero
  MATLAB Function : MATLAB Function  TreatAsAtomicUnit=on
  "MATLAB Function-freq=22 " : MATLAB Function  TreatAsAtomicUnit=on
  MATLAB Function-freq=24 : MATLAB Function  TreatAsAtomicUnit=on
  "MATLAB Function-freq=26 " : MATLAB Function  TreatAsAtomicUnit=on
  "MATLAB Function-freq=26-o " : MATLAB Function  TreatAsAtomicUnit=on
  "MATLAB Function1-freq=20 " : MATLAB Function  TreatAsAtomicUnit=on
  Memory : Memory  InheritSampleTime=on
  Memory1 : Memory  InheritSampleTime=on
  Mux : Mux  Inputs=2
  ODE : Subsystem
  Random Number1 : RandomNumber  SampleTime=20.2
  Step : Step  Time=52  Before=1  After=0  SampleTime=1
  Sum : Sum  Inputs=|++++
  Switch3 : Switch  Criteria=u2 > Threshold
  Switch4 : Switch  Criteria=u2 > Threshold
  Switch5 : Switch  Criteria=u2 > Threshold
  v : Outport
  q : Outport  Port=2
  Output : Outport  Port=3
  xy : Outport  Port=4
  wires:
  Memory1/1 -> Output/1
  Chart/4(Sense) -> Memory1/1
  Constant10/1 -> Switch5/1
  Constant9/1 -> ?
  [d0] -> ODE/3(d0)
  Chart/2(vreset) -> ODE/2(vreset)
  Constant8/1 -> Switch3/1
  Compare To Constant3/1 -> Chart/9(b)
  Switch3/1 -> q/1
  Memory/1 -> Switch3/3, ODE/1(q)
  Constant13/1 -> Switch4/1
  Switch5/1 -> Chart/2(gv)
  Chart/1(q) -> Memory/1
  [d2i] -> Chart/8(d2i)
  [VF] -> Chart/7(VF)
  ODE/1(vt_0) -> Switch4/3
  Add1/1 -> Switch5/3
  Constant14/1 -> Compare To Constant2/1
  Chart/3(d2) -> ODE/5(d2)
  [VR] -> Chart/6(VR)
  [Vm] -> Chart/5(Vm)
  [VT] -> Chart/4(VT)
  Chart/5(reset) -> ODE/7(reset)
  [d1] -> ODE/4(d1)
  [d3] -> ODE/6(d3)
  Switch4/1 -> v/1, Chart/1(v)
  Constant7/1 -> Switch3/2, Switch4/2, Switch5/2, Compare To Constant3/1
  Divide4/1 -> Sum/3
  gv4/1 -> Add4/1
  Divide5/1 -> Sum/4
  Constant6/1 -> Divide5/2
  Add4/1 -> Divide5/1
  Divide2/1 -> Add/2, Add2/2, Add3/2, Add4/2
  gv3/1 -> Add3/1
  Constant5/1 -> Divide4/2
  Add3/1 -> Divide4/1
  Sum/1 -> Add1/2
  Add2/1 -> Divide3/1
  Divide3/1 -> Sum/2
  Constant4/1 -> Divide3/2
  gv2/1 -> Add2/1
  Constant3/1 -> ?
  Add/1 -> Divide1/1
  Constant1/1 -> Divide2/2
  pulse/1 -> Add1/1
  Constant2/1 -> Divide1/2
  vin/1 -> Divide2/1
  Divide1/1 -> Sum/1
  gv1/1 -> Add/1
  [y] -> Mux/2
  Mux/1 -> xy/1
  [x] -> Mux/1
  "cfg "/1 -> Demux/1
  Demux/7 -> [VR]
  Demux/5 -> [VT]
  Demux/3 -> [d2i]
  Demux/4 -> [d3]
  Demux/10 -> [y]
  Demux/1 -> [d0]
  Demux/6 -> [Vm]
  Demux/9 -> [x]
  Demux/8 -> [VF]
  Demux/2 -> [d1]

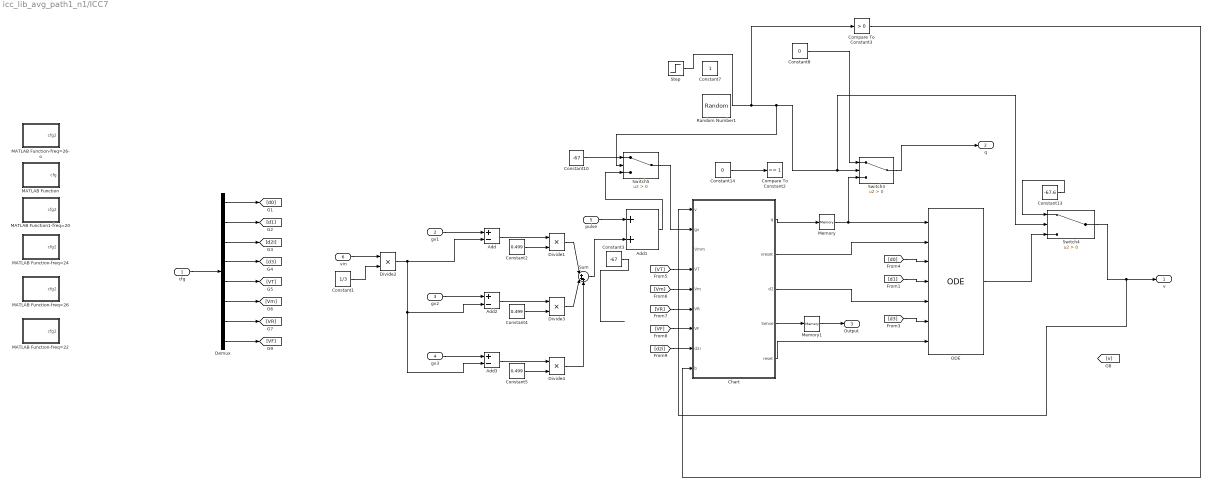
== system icc_lib_avg_path1_n1/ICC7 ==
  "cfg " : Inport
  gv1 : Inport  Port=2
  gv2 : Inport  Port=3
  gv3 : Inport  Port=4
  pulse : Inport  Port=5
  vin : Inport  Port=6
  Add : Sum  Inputs=+-
  Add1 : Sum
  Add2 : Sum  Inputs=+-
  Add3 : Sum  Inputs=+-
  Chart : Stateflow chart  TreatAsAtomicUnit=on
  Compare To Constant2 : simulink/Logic and Bit Operations/Compare To Constant  relop===  const=1  OutDataTypeStr=boolean
  Compare To Constant3 : simulink/Logic and Bit Operations/Compare To Constant  relop=>  const=0  OutDataTypeStr=boolean
  Constant1 : Constant  Value=1/3
  Constant10 : Constant  Value=-67
  Constant13 : Constant  Value=-67.6
  Constant14 : Constant  Value=0
  Constant2 : Constant  Value=0.499
  Constant3 : Constant  Value=-67
  Constant4 : Constant  Value=0.499
  Constant5 : Constant  Value=0.499
  Constant7 : Constant
  Constant8 : Constant  Value=0
  Demux : Demux  Outputs=8
  Divide{1..4} (4 alike) : Product  CollapseMode=Specified dimension  CollapseDim=2  SaturateOnIntegerOverflow=on  RndMeth=Zero
  MATLAB Function : MATLAB Function  TreatAsAtomicUnit=on
  "MATLAB Function-freq=22 " : MATLAB Function  TreatAsAtomicUnit=on
  MATLAB Function-freq=24 : MATLAB Function  TreatAsAtomicUnit=on
  "MATLAB Function-freq=26 " : MATLAB Function  TreatAsAtomicUnit=on
  "MATLAB Function-freq=26-o " : MATLAB Function  TreatAsAtomicUnit=on
  "MATLAB Function1-freq=20 " : MATLAB Function  TreatAsAtomicUnit=on
  Memory : Memory  InheritSampleTime=on
  Memory1 : Memory  InheritSampleTime=on
  ODE : $bdroot/ICC6/ODE  SystemSampleTime=-1
  Random Number1 : RandomNumber  SampleTime=20.2
  Step : Step  Time=52  Before=1  After=0  SampleTime=1
  Sum : Sum  Inputs=|+++
  Switch3 : Switch  Criteria=u2 > Threshold
  Switch4 : Switch  Criteria=u2 > Threshold
  Switch5 : Switch  Criteria=u2 > Threshold
  v : Outport
  q : Outport  Port=2
  Output : Outport  Port=3
  wires:
  Constant5/1 -> Divide4/2
  Constant4/1 -> Divide3/2
  Divide4/1 -> Sum/3
  Add2/1 -> Divide3/1
  Demux/3 -> [d2i]
  gv2/1 -> Add2/1
  Demux/4 -> [d3]
  Demux/1 -> [d0]
  Add/1 -> Divide1/1
  Constant2/1 -> Divide1/2
  vin/1 -> Divide2/1
  Add3/1 -> Divide4/1
  Constant1/1 -> Divide2/2
  gv3/1 -> Add3/1
  Divide1/1 -> Sum/1
  Divide3/1 -> Sum/2
  Divide2/1 -> Add2/2, Add3/2, Add/2
  gv1/1 -> Add/1
  Demux/5 -> [VT]
  Demux/8 -> [VF]
  "cfg "/1 -> Demux/1
  Demux/7 -> [VR]
  Demux/2 -> [d1]
  Demux/6 -> [Vm]
  [VF] -> Chart/7(VF)
  Constant8/1 -> Switch3/1
  Chart/4(Sense) -> Memory1/1
  Constant13/1 -> Switch4/1
  Switch3/1 -> q/1
  Constant10/1 -> Switch5/1
  Constant3/1 -> ?
  Chart/2(vreset) -> ODE/2
  Chart/3(d2) -> ODE/5
  Constant14/1 -> Compare To Constant2/1
  Memory/1 -> ODE/1, Switch3/3
  Compare To Constant3/1 -> Chart/9(b)
  [VR] -> Chart/6(VR)
  [d2i] -> Chart/8(d2i)
  Chart/1(q) -> Memory/1
  Memory1/1 -> Output/1
  pulse/1 -> Add1/1
  [VT] -> Chart/4(VT)
  Add1/1 -> Switch5/3
  ODE/1 -> Switch4/3
  [Vm] -> Chart/5(Vm)
  [d3] -> ODE/6
  Chart/5(reset) -> ODE/7
  [d1] -> ODE/4
  Switch4/1 -> Chart/1(v), v/1
  Switch5/1 -> Chart/2(gv)
  [d0] -> ODE/3
  Step/1 -> Compare To Constant3/1, Switch5/2, Switch4/2, Switch3/2
  Sum/1 -> Add1/2

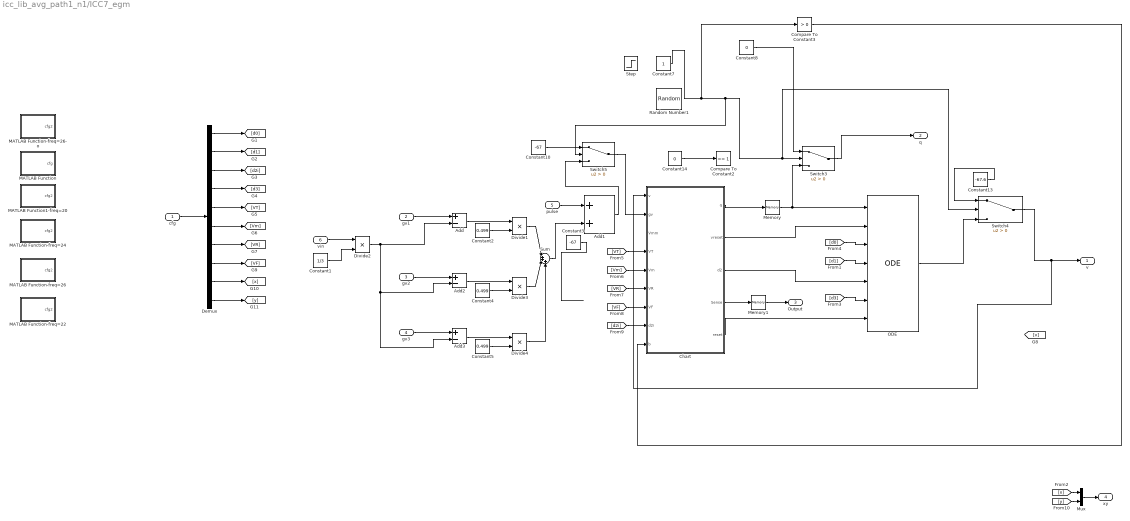
== system icc_lib_avg_path1_n1/ICC7_egm ==
  "cfg " : Inport
  gv1 : Inport  Port=2
  gv2 : Inport  Port=3
  gv3 : Inport  Port=4
  pulse : Inport  Port=5
  vin : Inport  Port=6
  Add : Sum  Inputs=+-
  Add1 : Sum
  Add2 : Sum  Inputs=+-
  Add3 : Sum  Inputs=+-
  Chart : Stateflow chart  TreatAsAtomicUnit=on
  Compare To Constant2 : simulink/Logic and Bit Operations/Compare To Constant  relop===  const=1  OutDataTypeStr=boolean
  Compare To Constant3 : simulink/Logic and Bit Operations/Compare To Constant  relop=>  const=0  OutDataTypeStr=boolean
  Constant1 : Constant  Value=1/3
  Constant10 : Constant  Value=-67
  Constant13 : Constant  Value=-67.6
  Constant14 : Constant  Value=0
  Constant2 : Constant  Value=0.499
  Constant3 : Constant  Value=-67
  Constant4 : Constant  Value=0.499
  Constant5 : Constant  Value=0.499
  Constant7 : Constant
  Constant8 : Constant  Value=0
  Demux : Demux  Outputs=10
  Divide{1..4} (4 alike) : Product  CollapseMode=Specified dimension  CollapseDim=2  SaturateOnIntegerOverflow=on  RndMeth=Zero
  MATLAB Function : MATLAB Function  TreatAsAtomicUnit=on
  "MATLAB Function-freq=22 " : MATLAB Function  TreatAsAtomicUnit=on
  MATLAB Function-freq=24 : MATLAB Function  TreatAsAtomicUnit=on
  "MATLAB Function-freq=26 " : MATLAB Function  TreatAsAtomicUnit=on
  "MATLAB Function-freq=26-o " : MATLAB Function  TreatAsAtomicUnit=on
  "MATLAB Function1-freq=20 " : MATLAB Function  TreatAsAtomicUnit=on
  Memory : Memory  InheritSampleTime=on
  Memory1 : Memory  InheritSampleTime=on
  Mux : Mux  Inputs=2
  ODE : $bdroot/ICC6/ODE  SystemSampleTime=-1
  Random Number1 : RandomNumber  SampleTime=20.2
  Step : Step  Time=52  Before=1  After=0  SampleTime=1
  Sum : Sum  Inputs=|+++
  Switch3 : Switch  Criteria=u2 > Threshold
  Switch4 : Switch  Criteria=u2 > Threshold
  Switch5 : Switch  Criteria=u2 > Threshold
  v : Outport
  q : Outport  Port=2
  Output : Outport  Port=3
  xy : Outport  Port=4
  wires:
  Sum/1 -> Add1/2
  Constant7/1 -> Switch3/2, Switch4/2, Switch5/2, Compare To Constant3/1
  [d0] -> ODE/3
  Switch5/1 -> Chart/2(gv)
  Switch4/1 -> v/1, Chart/1(v)
  [d1] -> ODE/4
  Chart/5(reset) -> ODE/7
  [d3] -> ODE/6
  [Vm] -> Chart/5(Vm)
  ODE/1 -> Switch4/3
  Add1/1 -> Switch5/3
  [VT] -> Chart/4(VT)
  pulse/1 -> Add1/1
  Memory1/1 -> Output/1
  Chart/1(q) -> Memory/1
  [d2i] -> Chart/8(d2i)
  [VR] -> Chart/6(VR)
  Compare To Constant3/1 -> Chart/9(b)
  Memory/1 -> Switch3/3, ODE/1
  Constant14/1 -> Compare To Constant2/1
  Chart/3(d2) -> ODE/5
  Chart/2(vreset) -> ODE/2
  Constant3/1 -> ?
  Constant10/1 -> Switch5/1
  Switch3/1 -> q/1
  Constant13/1 -> Switch4/1
  Chart/4(Sense) -> Memory1/1
  Constant8/1 -> Switch3/1
  [VF] -> Chart/7(VF)
  gv1/1 -> Add/1
  Divide2/1 -> Add/2, Add3/2, Add2/2
  Divide3/1 -> Sum/2
  Divide1/1 -> Sum/1
  gv3/1 -> Add3/1
  Constant1/1 -> Divide2/2
  Add3/1 -> Divide4/1
  vin/1 -> Divide2/1
  Constant2/1 -> Divide1/2
  Add/1 -> Divide1/1
  gv2/1 -> Add2/1
  Add2/1 -> Divide3/1
  Divide4/1 -> Sum/3
  Constant4/1 -> Divide3/2
  Constant5/1 -> Divide4/2
  Demux/3 -> [d2i]
  Demux/4 -> [d3]
  Demux/8 -> [VF]
  Demux/2 -> [d1]
  Demux/6 -> [Vm]
  Demux/7 -> [VR]
  Demux/1 -> [d0]
  "cfg "/1 -> Demux/1
  Demux/10 -> [y]
  Demux/9 -> [x]
  Demux/5 -> [VT]
  [y] -> Mux/2
  Mux/1 -> xy/1
  [x] -> Mux/1

== system icc_lib_avg_path1_n1/Subsystem ==
  Sense : Inport
  Chart : Stateflow chart  TreatAsAtomicUnit=on
  pace : Outport
  wires:
  Sense/1 -> Chart/1(Sense)
  Chart/1(pace) -> pace/1

== system icc_lib_avg_path1_n1/path ==
  mode1 : Inport
  mode2 : Inport  Port=2
  v1 : Inport  Port=3
  v2 : Inport  Port=4
  Data Type Conversion : DataTypeConversion  OutDataTypeStr=boolean
  Data Type Conversion1 : DataTypeConversion  OutDataTypeStr=boolean
  Delayed v1 : TransportDelay  DelayTime=0.1  BufferSize=200704
  Delayed v2 : TransportDelay  DelayTime=0.1  BufferSize=200704
  Logical Operator1 : Logic  Operator=OR  AllPortsSameDT=off  OutDataTypeStr=boolean
  Logical Operator2 : Logic  Operator=OR  AllPortsSameDT=off  OutDataTypeStr=boolean
  Path : Stateflow chart  TreatAsAtomicUnit=on
  Relay switch1 : MultiPortSwitch  DataPortOrder=Zero-based contiguous  Inputs=2  zeroidx=on
  Relay switch2 : MultiPortSwitch  DataPortOrder=Zero-based contiguous  Inputs=2  zeroidx=on
  S-R Flip-Flop : simulink_extras/Flip Flops/S-R Flip-Flop  initial_condition=0
  S-R Flip-Flop1 : simulink_extras/Flip Flops/S-R Flip-Flop  initial_condition=0
  Terminator : Terminator
  Terminator1 : Terminator
  Transport Delay1 : TransportDelay  DelayTime=0.1
  Transport Delay2 : TransportDelay  DelayTime=0.1
  cell1 resting : simulink/Logic and Bit Operations/Compare To Constant  relop===  const=0  OutDataTypeStr=boolean
  cell1FinishR : simulink/Logic and Bit Operations/Compare To Constant  relop=>=  const=2  OutDataTypeStr=boolean
  cell2 resting : simulink/Logic and Bit Operations/Compare To Constant  relop===  const=0  OutDataTypeStr=boolean
  cell2FinishR : simulink/Logic and Bit Operations/Compare To Constant  relop=>=  const=2  OutDataTypeStr=boolean
  zero : Constant  Value=0
  zero1 : Constant  Value=0
  relay_1 : Outport
  relay_2 : Outport  Port=2
  wires:
  Transport Delay1/1 -> cell1 resting/1, Path/2(mdelay1)
  mode2/1 -> Transport Delay2/1, cell2FinishR/1, Path/3(mode2)
  Delayed v2/1 -> Relay switch2/3
  Relay switch1/1 -> relay_1/1
  S-R Flip-Flop/1 -> Relay switch1/1
  S-R Flip-Flop/2 -> Terminator/1
  zero/1 -> Relay switch1/2
  zero1/1 -> Relay switch2/2
  v2/1 -> Delayed v2/1
  Path/2(relay2) -> Data Type Conversion1/1
  S-R Flip-Flop1/1 -> Relay switch2/1
  Delayed v1/1 -> Relay switch1/3
  Path/1(relay1) -> Data Type Conversion/1
  v1/1 -> Delayed v1/1
  S-R Flip-Flop1/2 -> Terminator1/1
  Relay switch2/1 -> relay_2/1
  Logical Operator1/1 -> S-R Flip-Flop/2
  cell2FinishR/1 -> Logical Operator1/1
  cell1 resting/1 -> Logical Operator1/2
  cell2 resting/1 -> Logical Operator2/2
  Logical Operator2/1 -> S-R Flip-Flop1/2
  cell1FinishR/1 -> Logical Operator2/1
  Transport Delay2/1 -> cell2 resting/1, Path/4(mdelay2)
  mode1/1 -> Path/1(mode1), Transport Delay1/1, cell1FinishR/1
  Data Type Conversion/1 -> S-R Flip-Flop/1
  Data Type Conversion1/1 -> S-R Flip-Flop1/1

== system icc_lib_avg_path1_n1/path1-2 ==
  mode1 : Inport
  mode2 : Inport  Port=2
  v1 : Inport  Port=3
  v2 : Inport  Port=4
  AND : Logic  IconShape=distinctive  AllPortsSameDT=off  OutDataTypeStr=boolean
  Data Type Conversion : DataTypeConversion  OutDataTypeStr=boolean
  Data Type Conversion1 : DataTypeConversion  OutDataTypeStr=boolean
  Delayed v1 : TransportDelay  DelayTime=0.5  BufferSize=200704
  Delayed v2 : TransportDelay  DelayTime=0.5  BufferSize=200704
  Logical Operator1 : Logic  Operator=OR  AllPortsSameDT=off  OutDataTypeStr=boolean
  Logical Operator2 : Logic  Operator=OR  AllPortsSameDT=off  OutDataTypeStr=boolean
  Path : Stateflow chart  TreatAsAtomicUnit=on
  Relay switch1 : MultiPortSwitch  DataPortOrder=Zero-based contiguous  Inputs=2  zeroidx=on
  Relay switch2 : MultiPortSwitch  DataPortOrder=Zero-based contiguous  Inputs=2  zeroidx=on
  S-R Flip-Flop : simulink_extras/Flip Flops/S-R Flip-Flop  initial_condition=0
  S-R Flip-Flop1 : simulink_extras/Flip Flops/S-R Flip-Flop  initial_condition=0
  Terminator : Terminator
  Terminator1 : Terminator
  Transport Delay1 : TransportDelay  DelayTime=0.1
  Transport Delay2 : TransportDelay  DelayTime=0.1
  cell1 resting : simulink/Logic and Bit Operations/Compare To Constant  relop===  const=0  OutDataTypeStr=boolean
  cell1FinishR : simulink/Logic and Bit Operations/Compare To Constant  relop=>=  const=1  OutDataTypeStr=boolean
  cell2 resting : simulink/Logic and Bit Operations/Compare To Constant  relop===  const=0  OutDataTypeStr=boolean
  cell2FinishR : simulink/Logic and Bit Operations/Compare To Constant  relop=>=  const=1  OutDataTypeStr=boolean
  cell2FinishR1 : simulink/Logic and Bit Operations/Compare To Constant  relop=~=  const=0  OutDataTypeStr=boolean
  cell2FinishR2 : simulink/Logic and Bit Operations/Compare To Constant  relop=~=  const=4  OutDataTypeStr=boolean
  zero : Constant  Value=-67.6
  zero1 : Constant  Value=-67.6
  relay_1 : Outport
  relay_2 : Outport  Port=2
  wires:
  cell2FinishR2/1 -> AND/1
  cell2FinishR1/1 -> AND/2
  Transport Delay1/1 -> cell1 resting/1, Path/2(mdelay1)
  mode2/1 -> Transport Delay2/1, Path/3(mode2), cell2FinishR1/1, cell2FinishR2/1
  Delayed v2/1 -> Relay switch2/3
  Relay switch1/1 -> relay_1/1
  S-R Flip-Flop/1 -> Relay switch1/1
  S-R Flip-Flop/2 -> Terminator/1
  zero/1 -> Relay switch1/2
  zero1/1 -> Relay switch2/2
  v2/1 -> Delayed v2/1
  Path/2(relay2) -> Data Type Conversion1/1
  S-R Flip-Flop1/1 -> Relay switch2/1
  Delayed v1/1 -> Relay switch1/3
  Path/1(relay1) -> Data Type Conversion/1
  v1/1 -> Delayed v1/1
  S-R Flip-Flop1/2 -> Terminator1/1
  Relay switch2/1 -> relay_2/1
  Logical Operator1/1 -> S-R Flip-Flop/2
  AND/1 -> Logical Operator1/1
  cell1 resting/1 -> Logical Operator1/2
  cell2 resting/1 -> Logical Operator2/2
  Logical Operator2/1 -> S-R Flip-Flop1/2
  cell1FinishR/1 -> Logical Operator2/1
  Transport Delay2/1 -> cell2 resting/1, Path/4(mdelay2)
  mode1/1 -> Path/1(mode1), Transport Delay1/1, cell1FinishR/1
  Data Type Conversion/1 -> S-R Flip-Flop/1
  Data Type Conversion1/1 -> S-R Flip-Flop1/1

== system icc_lib_avg_path1_n1/path_EGM ==
  mode1 : Inport
  mode2 : Inport  Port=2
  v1 : Inport  Port=3
  v2 : Inport  Port=4
  "xy1 " : Inport  Port=5
  xy2 : Inport  Port=6
  AND : Logic  IconShape=distinctive  AllPortsSameDT=off  OutDataTypeStr=boolean
  Data Type Conversion : DataTypeConversion  OutDataTypeStr=boolean
  Data Type Conversion1 : DataTypeConversion  OutDataTypeStr=boolean
  Delayed v1 : TransportDelay  DelayTime=0.1  BufferSize=200704
  Delayed v2 : TransportDelay  DelayTime=0.1  BufferSize=200704
  Demux : Demux  Outputs=2
  Demux1 : Demux  Outputs=2
  Logical Operator1 : Logic  Operator=OR  AllPortsSameDT=off  OutDataTypeStr=boolean
  Logical Operator2 : Logic  Operator=OR  AllPortsSameDT=off  OutDataTypeStr=boolean
  Mux : Mux  Inputs=6
  Path : Stateflow chart  TreatAsAtomicUnit=on
  Relay switch1 : MultiPortSwitch  DataPortOrder=Zero-based contiguous  Inputs=2  zeroidx=on
  Relay switch2 : MultiPortSwitch  DataPortOrder=Zero-based contiguous  Inputs=2  zeroidx=on
  S-R Flip-Flop : simulink_extras/Flip Flops/S-R Flip-Flop  initial_condition=0
  S-R Flip-Flop1 : simulink_extras/Flip Flops/S-R Flip-Flop  initial_condition=0
  Terminator : Terminator
  Terminator1 : Terminator
  Transport Delay1 : TransportDelay  DelayTime=0.1
  Transport Delay2 : TransportDelay  DelayTime=0.1
  cell1 resting : simulink/Logic and Bit Operations/Compare To Constant  relop===  const=0  OutDataTypeStr=boolean
  cell1FinishR : simulink/Logic and Bit Operations/Compare To Constant  relop=>=  const=1  OutDataTypeStr=boolean
  cell2 resting : simulink/Logic and Bit Operations/Compare To Constant  relop===  const=0  OutDataTypeStr=boolean
  cell2FinishR : simulink/Logic and Bit Operations/Compare To Constant  relop=>=  const=1  OutDataTypeStr=boolean
  cell2FinishR1 : simulink/Logic and Bit Operations/Compare To Constant  relop=~=  const=0  OutDataTypeStr=boolean
  cell2FinishR2 : simulink/Logic and Bit Operations/Compare To Constant  relop=~=  const=4  OutDataTypeStr=boolean
  zero : Constant  Value=-67.6
  zero1 : Constant  Value=-67.6
  relay_1 : Outport
  relay_2 : Outport  Port=2
  egm : Outport  Port=3
  wires:
  Data Type Conversion1/1 -> S-R Flip-Flop1/1
  Data Type Conversion/1 -> S-R Flip-Flop/1
  mode1/1 -> cell1FinishR/1, Transport Delay1/1, Path/1(mode1)
  Transport Delay2/1 -> Path/4(mdelay2), cell2 resting/1
  cell1FinishR/1 -> Logical Operator2/1
  Logical Operator2/1 -> S-R Flip-Flop1/2
  cell2 resting/1 -> Logical Operator2/2
  cell1 resting/1 -> Logical Operator1/2
  AND/1 -> Logical Operator1/1
  Logical Operator1/1 -> S-R Flip-Flop/2
  Relay switch2/1 -> relay_2/1
  S-R Flip-Flop1/2 -> Terminator1/1
  v1/1 -> Delayed v1/1
  Path/1(relay1) -> Data Type Conversion/1
  Delayed v1/1 -> Relay switch1/3
  S-R Flip-Flop1/1 -> Relay switch2/1
  Path/2(relay2) -> Data Type Conversion1/1
  v2/1 -> Delayed v2/1
  zero1/1 -> Relay switch2/2
  zero/1 -> Relay switch1/2
  S-R Flip-Flop/2 -> Terminator/1
  S-R Flip-Flop/1 -> Relay switch1/1
  Relay switch1/1 -> relay_1/1
  Delayed v2/1 -> Relay switch2/3
  mode2/1 -> cell2FinishR2/1, cell2FinishR1/1, Path/3(mode2), Transport Delay2/1
  Transport Delay1/1 -> Path/2(mdelay1), cell1 resting/1
  cell2FinishR1/1 -> AND/2
  cell2FinishR2/1 -> AND/1
  "xy1 "/1 -> Demux/1
  Demux/1 -> [x1]
  Demux/2 -> [y1]
  Mux/1 -> egm/1
  Path/3(t1) -> [t1]
  Path/4(t2) -> [t2]
  [t1] -> Mux/1
  [t2] -> Mux/2
  [x1] -> Mux/3
  [y1] -> Mux/4
  xy2/1 -> Demux1/1
  Demux1/1 -> [x2]
  Demux1/2 -> [y2]
  [y2] -> Mux/6
  [x2] -> Mux/5
